simulink model "Fazy"  (R2024b)
settings: Solver=VariableStepAuto  StartTime=0.0  StopTime=1000.0  RelTol=1e-3
values from neighbouring files (symbols this model uses):
  bX = 1    [Lab5.m]
  ddx = 1    [Lab5.m]
  dx = 1    [Lab5.m]
  W = 0.01    [Lab5.m]
  X = 1    [Lab5.m]
settings Model: Creator=pawli  LastModifiedBy=pawli

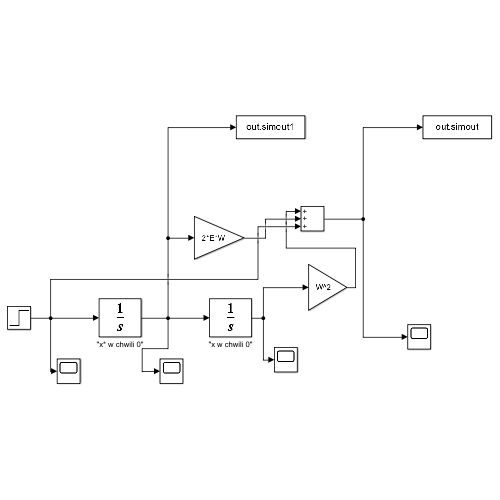
[thumbnail: Simulink's stored preview of the top-level diagram]
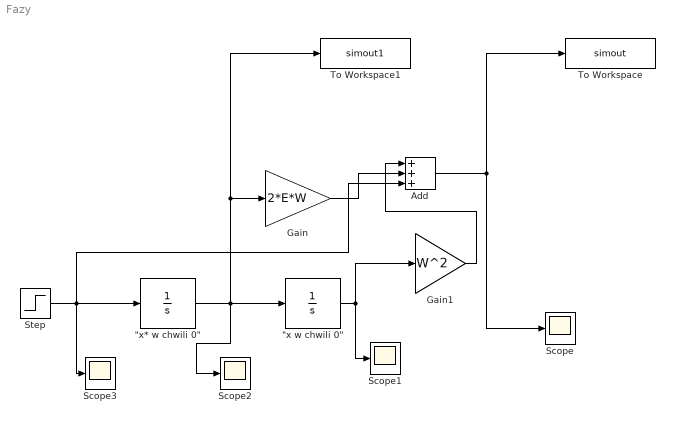
== system Fazy ==
  "\"x w chwili 0\"" : Integrator  InitialCondition=ddx
  "\"x* w chwili 0\"" : Integrator  InitialCondition=dx
  Add : Sum  Inputs=+++
  Gain : Gain  Gain=2*E*W
  Gain1 : Gain  Gain=W^2
  Scope{,1..3} (4 alike) : Scope
  Step : Step  Time=300  Before=X  After=X+bX  SampleTime=0
  To Workspace : ToWorkspace  VariableName=simout  SampleTime=-1
  To Workspace1 : ToWorkspace  VariableName=simout1  SampleTime=-1
  wires:
  Step/1 -> Scope3/1, Add/3, "\"x* w chwili 0\""/1
  "\"x w chwili 0\""/1 -> Scope1/1, Gain1/1
  Gain1/1 -> Add/1
  Gain/1 -> Add/2
  Add/1 -> Scope/1, To Workspace/1
  "\"x* w chwili 0\""/1 -> "\"x w chwili 0\""/1, Gain/1, To Workspace1/1, Scope2/1
